simulink model "motor"  (R2024b)
settings: Solver=VariableStepAuto  StartTime=0.0  StopTime=100.0  RelTol=1e-3
values from neighbouring files (symbols this model uses):
  Gp = K/(T1*s*(T2*s+1))    [main.m]
  Kd = 0    [Z_N1.m]
  Ki = 0    [Z_N1.m]
  Kp = 0    [Z_N1.m]
settings Model: Creator=egoru  LastModifiedBy=tolst

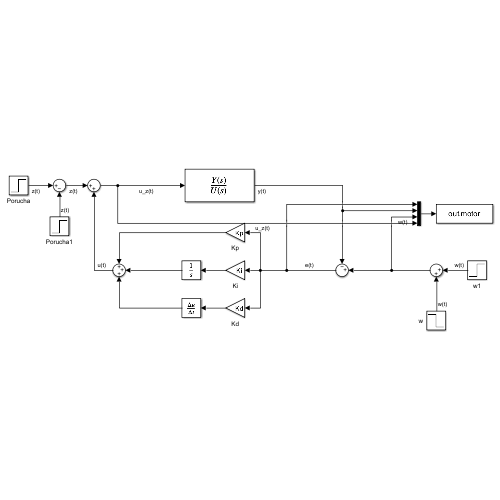
[thumbnail: Simulink's stored preview of the top-level diagram]
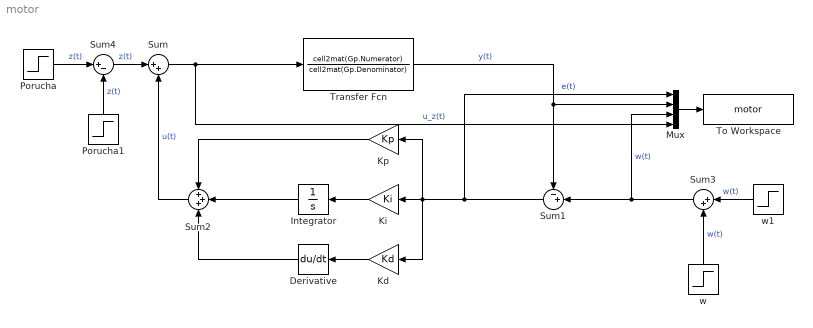
== system motor ==
  Derivative : Derivative
  Integrator : Integrator
  Kd : Gain  Gain=Kd
  Ki : Gain  Gain=Ki
  Kp : Gain  Gain=Kp
  Mux : Mux
  Porucha : Step  Time=40  After=0.2  SampleTime=0
  Porucha1 : Step  Time=50  After=0.2  SampleTime=0
  Sum : Sum  Inputs=|++
  Sum1 : Sum  Inputs=-+|
  Sum2 : Sum  Inputs=+++
  Sum3 : Sum  Inputs=|++
  Sum4 : Sum  Inputs=|+-
  To Workspace : ToWorkspace  VariableName=motor  SaveFormat=Timeseries  SampleTime=-1
  Transfer Fcn : TransferFcn  Numerator=cell2mat(Gp.Numerator)  Denominator=cell2mat(Gp.Denominator)
  w : Step  Time=70  After=-0.2  SampleTime=0
  w1 : Step  Time=10  SampleTime=0
  wires:
  Sum3/1 -> Mux/3, Sum1/2  "w(t)"
  Transfer Fcn/1 -> Mux/2, Sum1/1  "y(t)"
  Sum/1 -> Mux/4, Transfer Fcn/1  "u_z(t)"
  Sum2/1 -> Sum/2  "u(t)"
  Sum1/1 -> Mux/1, Kd/1, Ki/1, Kp/1  "e(t)"
  Mux/1 -> To Workspace/1
  Integrator/1 -> Sum2/2
  Ki/1 -> Integrator/1
  Derivative/1 -> Sum2/3
  Kd/1 -> Derivative/1
  Kp/1 -> Sum2/1
  w/1 -> Sum3/2  "w(t)"
  w1/1 -> Sum3/1  "w(t)"
  Porucha1/1 -> Sum4/2  "z(t)"
  Porucha/1 -> Sum4/1  "z(t)"
  Sum4/1 -> Sum/1  "z(t)"
